simulink model "ABS_Controller"  (R2024b)
settings: Solver=FixedStepDiscrete  StartTime=0.0  StopTime=10  FixedStep=0.0001  RelTol=1e-3
settings Model: Creator=devap  LastModifiedBy=devap
settings DataIOCC: SaveOutput=off  SaveTime=off
settings OptimizationCC: DefaultParameterBehavior=Inlined  EnhancedBackFolding=on  PassReuseOutputArgsAs=Individual arguments  ZeroExternalMemoryAtStartup=off  ZeroInternalMemoryAtStartup=off  OptimizeBlockOrder=speed  DifferentSizesBufferReuse=on  OptimizationCustomize=off  EfficientTunableParamExpr=on
settings DebuggingCC: ParameterTunabilityLossMsg=error  UnderSpecifiedDimensionMsg=warning
settings SFSimCC: MATLABDynamicMemAlloc=off
settings RTWCC: Description=Embedded Coder  SystemTargetFile=ert.tlc  TemplateMakefile=ert_default_tmf
settings CodeAppCC: ForceParamTrailComments=on  IgnoreCustomStorageClasses=off  OperatorAnnotations=on  SimulinkDataObjDesc=on  SFDataObjDesc=on  InsertBlockDesc=on
settings ERTTargetCC: TargetLangStandard=C99 (ISO)  GenerateSampleERTMain=on  CombineOutputUpdateFcns=off  ERTCustomFileTemplate=example_file_process.tlc

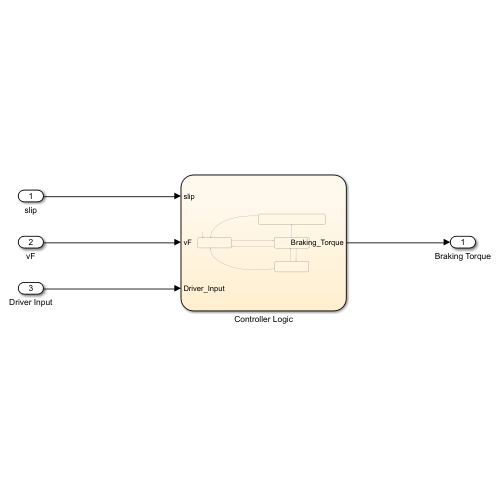
[thumbnail: Simulink's stored preview of the top-level diagram]
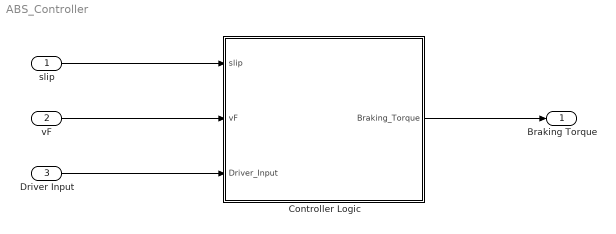
== system ABS_Controller ==
  slip : Inport  OutDataTypeStr=double  PortDimensions=1
  vF : Inport  Port=2  OutDataTypeStr=double  PortDimensions=1
  Driver Input : Inport  Port=3  OutDataTypeStr=double  PortDimensions=1
  Controller Logic : Stateflow chart  TreatAsAtomicUnit=on  SystemSampleTime=0.0001
      settings: PortSchema="{\"entries\":[{\"content\":{\"sides\":[{\"content\":{},\"type\":\"ConnectorPlacement.EquallySpacedRectSide\",\"uuid\":\"21f18844-d46f-4192-8888-e19f26fc3edc\"},{\"content\":{\"side\":\"RIGHT\"},\"type\":\"ConnectorPlacement.EquallySpacedRectSide\",\"uuid\":\"7bd71700-bad4-4cbb-9483-04161d3aff77\"},{\"content\":{\"connectorIds\":[\"In3\",\"In2\",\"In1\"],\"side\":\"TOP\"},\"type\":\"ConnectorPlacement.EquallySpacedRectSide\",\"uuid\":\"4756a897-bcf0-41d1-bf8d-a96ee74f6ad2\"},{\"content\":{\"connectorIds\":[\"Out1\"],\"side\":\"BOTTOM\"},\"type\":\"ConnectorPlacement.EquallySpacedRectSide\",\"uuid\":\"313fe5f9-b121-4e9c-8752-7e0554df123c\"}]},\"type\":\"ConnectorPlacement.EquallySpacedConnector\",\"uuid\":\"67e74c9c-ac74-4bfd-968a-12aff3b01f59\"}],\"packageUris\":[\"http://schema.mathworks.com/mf0/Connector/R2020b\"],\"version\":\"1.0\"}"
  Braking Torque : Outport  OutDataTypeStr=double  PortDimensions=1  SampleTime=[0.0001,0]
  wires:
  slip/1 -> Controller Logic/1(slip)
  Controller Logic/1(Braking_Torque) -> Braking Torque/1
  Driver Input/1 -> Controller Logic/3(Driver_Input)
  vF/1 -> Controller Logic/2(vF)

== stateflow chart ABS_Controller/Controller Logic ==
  state Low_Torque
    entry: Braking_Torque=BT_max;
    during: Braking_Torque=min(Braking_Torque - step_size , BT_max);
  state Braking
    during: Braking_Torque=BT_max;
  state No_Braking
    during: Braking_Torque=0;
  state ABS_ON
    during: Braking_Torque=0;
  Low_Torque -> No_Braking : [Driver_Input == 0]
  Braking -> Low_Torque [order 3] : [vF <= 1.786]
  (default) -> No_Braking
  No_Braking -> Braking : [Driver_Input == 1]
  Braking -> No_Braking [order 2] : [Driver_Input == 0]
  ABS_ON -> No_Braking [order 2] : [Driver_Input == 0]
  ABS_ON -> Braking [order 1] : [Driver_Input == 1 && slip <= 0.13]
  Braking -> ABS_ON [order 1] : [Driver_Input == 1 && slip > 0.13]
  data: slip input; vF input; Driver_Input input; Braking_Torque output; BT_max parameter; step_size constant double =0.1
